simulink model "NoC_4x4x3"  (R2015a)
settings: Solver=ode45  StartTime=0.0  StopTime=10.0  RelTol=1e-3
undefined symbols (not defined in the file or in its folder): des, SELECT
undefined symbols (not defined in the file): MAX, MIN, T
libraries: simulink x48
(part 4 of 12)

== system NoC_4x4x3/Layer/PE00 ==
  Constant : Constant  Value=SELECT
  Create Generator Selection Variable : Subsystem  TreatAsAtomicUnit=on
      settings: PropExecContextOutsideSubsystem=on
  DST : EventBasedRandomNumber  Distribution=Arbitrary discrete  minUnid=1  maxUnid=16  numValueUnid=5  valueVecDisc=[1 2 3 4]  probVecDisc=[.25 .25 .25 .25]  Seed=SEED+5
  DST1 : EventBasedRandomNumber  Distribution=Arbitrary discrete  minUnid=1  maxUnid=16  numValueUnid=5  valueVecDisc=[1 2 3 4]  probVecDisc=[.25 .25 .25 .25]  Seed=SEED+50
  DST2 : EventBasedRandomNumber  Distribution=Arbitrary discrete  minUnid=1  maxUnid=16  numValueUnid=5  valueVecDisc=[1 2 3 4]  probVecDisc=[.25 .25 .25 .25]  Seed=SEED+500
  Enabled Gate : EnabledGate
  Entity Departure Event to Function-Call Event : EntityDepartureFunctionCallGenerator
  Entity Sink : EntitySink
  Entity Sink1 : EntitySink
  Generator 1 : TimeBasedEntityGenerator  Distribution=Exponential  Period=.1  InitialSeed=SEED+10  Maximum=.2  Mean=B  ResponseWhenUnblocked=Delayed restart  EntityType=Standard
  Infinite Server : InfiniteServer  ServiceTime=0  StatAverageWait=on
      settings: OutputPortMap=o4
  Input Switch : InputSwitch  SwitchingCriterion=From signal port p  StatNumberDeparted=on
  Loss : ToWorkspace  VariableName=Corner_Loss_Z2  SaveFormat=Timeseries  SampleTime=-1
  N : ToWorkspace  VariableName=Corner_N_Z2  SaveFormat=Timeseries  SampleTime=-1
  Read Timer : ReadTimer  TimerTag=Departure  StatAverageTimeElapsed=on
      settings: OutputPortMap=o3
  Router : ToWorkspace  VariableName=Corner_Mean_Z2  SaveFormat=Timeseries  SampleTime=-1
  Set Attribute : SetAttribute  AttributeName=DST_X|DST_Y|DST_Z  AttributeFrom=Signal port|Signal port|Signal port  AttributeValue=16|1|1  AttributeTreatAsVector=0|1|1  StatNumberDeparted=on  EvaluatedAttributeValue={ [];[];[]}
      settings: InputPortMap=u0,u1,u2
  Start Timer1 : StartTimer  TimerTag=Departure
  Time-Based Entity Generator : TimeBasedEntityGenerator  Distribution=Exponential  Period=15  InitialSeed=50510  Maximum=2  Mean=A  PriorityEntityGeneration=350  EntityType=Standard
  Time-Based Entity Generator1 : TimeBasedEntityGenerator  Period=REGULAR
  Time-Based Entity Generator2 : TimeBasedEntityGenerator  Distribution=Uniform  InitialSeed=56944  Minimum=MINU  Maximum=MAXU
  Data_out : PMIOPort  Port=1  Side=Right
  Data_in : PMIOPort  Port=2  Side=Left
  wires:
  Create Generator Selection Variable/1(Out1) -> Enabled Gate/1
  Entity Departure Event to Function-Call Event/1 -> Create Generator Selection Variable/Trigger
  Constant/1 -> Input Switch/1
  Read Timer/1 -> Router/1
  Input Switch/1 -> N/1
  DST/1 -> Set Attribute/1
  DST1/1 -> Set Attribute/2
  DST2/1 -> Set Attribute/3
  Infinite Server/1 -> Loss/1
  connections:
  Entity Departure Event to Function-Call Event/RConn1 -- Entity Sink/LConn1
  Time-Based Entity Generator/RConn1 -- Entity Departure Event to Function-Call Event/LConn1
  Generator 1/RConn1 -- Enabled Gate/LConn1
  Time-Based Entity Generator1/RConn1 -- Input Switch/LConn1
  Input Switch/LConn2 -- Time-Based Entity Generator2/RConn1
  Enabled Gate/RConn1 -- Input Switch/LConn3
  Start Timer1/LConn1 -- Set Attribute/RConn1
  Set Attribute/LConn1 -- Input Switch/RConn1
  Entity Sink1/LConn1 -- Read Timer/RConn1
  Data_in/RConn1 -- Read Timer/LConn1
  Start Timer1/RConn1 -- Infinite Server/LConn1
  Infinite Server/RConn1 -- Data_out/RConn1

== system NoC_4x4x3/Layer/PE01 ==
  Constant : Constant  Value=SELECT
  Create Generator Selection Variable : Subsystem  TreatAsAtomicUnit=on
      settings: PropExecContextOutsideSubsystem=on
  DST : EventBasedRandomNumber  Distribution=Arbitrary discrete  minUnid=1  maxUnid=16  numValueUnid=5  valueVecDisc=[1 2 3 4]  probVecDisc=[.25 .25 .25 .25]  Seed=SEED+5
  DST1 : EventBasedRandomNumber  Distribution=Arbitrary discrete  minUnid=1  maxUnid=16  numValueUnid=5  valueVecDisc=[1 2 3 4]  probVecDisc=[.25 .25 .25 .25]  Seed=SEED+50
  DST2 : EventBasedRandomNumber  Distribution=Arbitrary discrete  minUnid=1  maxUnid=16  numValueUnid=5  valueVecDisc=[1 2 3 4]  probVecDisc=[.25 .25 .25 .25]  Seed=SEED+500
  Enabled Gate : EnabledGate
  Entity Departure Event to Function-Call Event : EntityDepartureFunctionCallGenerator
  Entity Sink : EntitySink
  Entity Sink1 : EntitySink
  Generator 1 : TimeBasedEntityGenerator  Distribution=Exponential  Period=.1  InitialSeed=SEED+10  Maximum=.2  Mean=B  ResponseWhenUnblocked=Delayed restart  EntityType=Standard
  Infinite Server : InfiniteServer  ServiceTime=0  StatAverageWait=on
      settings: OutputPortMap=o4
  Input Switch : InputSwitch  SwitchingCriterion=From signal port p  StatNumberDeparted=on
  Loss : ToWorkspace  VariableName=Side_Loss_Z2  SaveFormat=Timeseries  SampleTime=-1
  N : ToWorkspace  VariableName=Side_N_Z2  SaveFormat=Timeseries  SampleTime=-1
  Read Timer : ReadTimer  TimerTag=Departure  StatAverageTimeElapsed=on
      settings: OutputPortMap=o3
  Router : ToWorkspace  VariableName=Side_Mean_Z2  SaveFormat=Timeseries  SampleTime=-1
  Set Attribute : SetAttribute  AttributeName=DST_X|DST_Y|DST_Z  AttributeFrom=Signal port|Signal port|Signal port  AttributeValue=16|1|1  AttributeTreatAsVector=0|1|1  StatNumberDeparted=on  EvaluatedAttributeValue={ [];[];[]}
      settings: InputPortMap=u0,u1,u2
  Start Timer : StartTimer  TimerTag=Departure
  Time-Based Entity Generator : TimeBasedEntityGenerator  Distribution=Exponential  Period=15  InitialSeed=60161  Maximum=2  Mean=A  PriorityEntityGeneration=350  EntityType=Standard
  Time-Based Entity Generator1 : TimeBasedEntityGenerator  Period=REGULAR
  Time-Based Entity Generator2 : TimeBasedEntityGenerator  Distribution=Uniform  InitialSeed=63378  Minimum=MINU  Maximum=MAXU
  Data_out : PMIOPort  Port=1  Side=Right
  Data_in : PMIOPort  Port=2  Side=Left
  wires:
  DST2/1 -> Set Attribute/3
  DST1/1 -> Set Attribute/2
  DST/1 -> Set Attribute/1
  Input Switch/1 -> N/1
  Read Timer/1 -> Router/1
  Constant/1 -> Input Switch/1
  Entity Departure Event to Function-Call Event/1 -> Create Generator Selection Variable/Trigger
  Create Generator Selection Variable/1(Out1) -> Enabled Gate/1
  Infinite Server/1 -> Loss/1
  connections:
  Data_in/RConn1 -- Read Timer/LConn1
  Entity Sink1/LConn1 -- Read Timer/RConn1
  Set Attribute/LConn1 -- Input Switch/RConn1
  Start Timer/LConn1 -- Set Attribute/RConn1
  Enabled Gate/RConn1 -- Input Switch/LConn3
  Input Switch/LConn2 -- Time-Based Entity Generator2/RConn1
  Time-Based Entity Generator1/RConn1 -- Input Switch/LConn1
  Generator 1/RConn1 -- Enabled Gate/LConn1
  Time-Based Entity Generator/RConn1 -- Entity Departure Event to Function-Call Event/LConn1
  Entity Departure Event to Function-Call Event/RConn1 -- Entity Sink/LConn1
  Start Timer/RConn1 -- Infinite Server/LConn1
  Infinite Server/RConn1 -- Data_out/RConn1

== system NoC_4x4x3/Layer/PE02 ==
  Cancel Timeout : CancelTimeout
  Constant : Constant  Value=SELECT
  Create Generator Selection Variable : Subsystem  TreatAsAtomicUnit=on
      settings: PropExecContextOutsideSubsystem=on
  DST : EventBasedRandomNumber  Distribution=Arbitrary discrete  minUnid=1  maxUnid=16  numValueUnid=5  valueVecDisc=[1 2 3 4]  probVecDisc=[.25 .25 .25 .25]  Seed=SEED+5
  DST1 : EventBasedRandomNumber  Distribution=Arbitrary discrete  minUnid=1  maxUnid=16  numValueUnid=5  valueVecDisc=[1 2 3 4]  probVecDisc=[.25 .25 .25 .25]  Seed=SEED+50
  DST2 : EventBasedRandomNumber  Distribution=Arbitrary discrete  minUnid=1  maxUnid=16  numValueUnid=5  valueVecDisc=[1 2 3 4]  probVecDisc=[.25 .25 .25 .25]  Seed=SEED+500
  Enabled Gate : EnabledGate
  Entity Departure Event to Function-Call Event : EntityDepartureFunctionCallGenerator
  Entity Sink : EntitySink
  Entity Sink1 : EntitySink
  Entity Sink2 : EntitySink
  Generator 1 : TimeBasedEntityGenerator  Distribution=Exponential  Period=.1  InitialSeed=SEED+10  Maximum=.2  Mean=B  ResponseWhenUnblocked=Delayed restart  EntityType=Standard
  Infinite Server : InfiniteServer  ServiceTime=D  EnableTOPort=on
  Input Switch : InputSwitch  SwitchingCriterion=From signal port p
  Schedule Timeout : ScheduleTimeout  TimeoutInterval=D
  Set Attribute : SetAttribute  AttributeName=DST_X|DST_Y|DST_Z  AttributeFrom=Signal port|Signal port|Signal port  AttributeValue=16|1|1  AttributeTreatAsVector=0|1|1  EvaluatedAttributeValue={ [];[];[]}
      settings: InputPortMap=u0,u1,u2
  Start Timer : StartTimer  TimerTag=Departure
  Time-Based Entity Generator : TimeBasedEntityGenerator  Distribution=Exponential  Period=15  InitialSeed=1059  Maximum=2  Mean=A  PriorityEntityGeneration=350  EntityType=Standard
  Time-Based Entity Generator1 : TimeBasedEntityGenerator  Period=REGULAR
  Time-Based Entity Generator2 : TimeBasedEntityGenerator  Distribution=Uniform  InitialSeed=4276  Minimum=MINU  Maximum=MAXU
  Data_out : PMIOPort  Port=1  Side=Right
  Data_in : PMIOPort  Port=2  Side=Left
  wires:
  DST2/1 -> Set Attribute/3
  DST1/1 -> Set Attribute/2
  DST/1 -> Set Attribute/1
  Constant/1 -> Input Switch/1
  Entity Departure Event to Function-Call Event/1 -> Create Generator Selection Variable/Trigger
  Create Generator Selection Variable/1(Out1) -> Enabled Gate/1
  connections:
  Infinite Server/RConn2 -- Entity Sink2/LConn1
  Schedule Timeout/RConn1 -- Infinite Server/LConn1
  Entity Sink1/LConn1 -- Data_in/RConn1
  Start Timer/LConn1 -- Cancel Timeout/RConn1
  Data_out/RConn1 -- Start Timer/RConn1
  Set Attribute/LConn1 -- Input Switch/RConn1
  Cancel Timeout/LConn1 -- Infinite Server/RConn1
  Schedule Timeout/LConn1 -- Set Attribute/RConn1
  Enabled Gate/RConn1 -- Input Switch/LConn3
  Input Switch/LConn2 -- Time-Based Entity Generator2/RConn1
  Time-Based Entity Generator1/RConn1 -- Input Switch/LConn1
  Generator 1/RConn1 -- Enabled Gate/LConn1
  Time-Based Entity Generator/RConn1 -- Entity Departure Event to Function-Call Event/LConn1
  Entity Departure Event to Function-Call Event/RConn1 -- Entity Sink/LConn1

== system NoC_4x4x3/Layer/PE03 ==
  Cancel Timeout : CancelTimeout
  Constant : Constant  Value=SELECT
  Create Generator Selection Variable : Subsystem  TreatAsAtomicUnit=on
      settings: PropExecContextOutsideSubsystem=on
  DST : EventBasedRandomNumber  Distribution=Arbitrary discrete  minUnid=1  maxUnid=16  numValueUnid=5  valueVecDisc=[1 2 3 4]  probVecDisc=[.25 .25 .25 .25]  Seed=SEED+5
  DST1 : EventBasedRandomNumber  Distribution=Arbitrary discrete  minUnid=1  maxUnid=16  numValueUnid=5  valueVecDisc=[1 2 3 4]  probVecDisc=[.25 .25 .25 .25]  Seed=SEED+50
  DST2 : EventBasedRandomNumber  Distribution=Arbitrary discrete  minUnid=1  maxUnid=16  numValueUnid=5  valueVecDisc=[1 2 3 4]  probVecDisc=[.25 .25 .25 .25]  Seed=SEED+500
  Enabled Gate : EnabledGate
  Entity Departure Event to Function-Call Event : EntityDepartureFunctionCallGenerator
  Entity Sink : EntitySink
  Entity Sink1 : EntitySink
  Entity Sink2 : EntitySink
  Generator 1 : TimeBasedEntityGenerator  Distribution=Exponential  Period=.1  InitialSeed=SEED+10  Maximum=.2  Mean=B  ResponseWhenUnblocked=Delayed restart  EntityType=Standard
  Infinite Server : InfiniteServer  ServiceTime=D  EnableTOPort=on
  Input Switch : InputSwitch  SwitchingCriterion=From signal port p
  Schedule Timeout : ScheduleTimeout  TimeoutInterval=D
  Set Attribute : SetAttribute  AttributeName=DST_X|DST_Y|DST_Z  AttributeFrom=Signal port|Signal port|Signal port  AttributeValue=16|1|1  AttributeTreatAsVector=0|1|1  EvaluatedAttributeValue={ [];[];[]}
      settings: InputPortMap=u0,u1,u2
  Start Timer : StartTimer  TimerTag=Departure
  Time-Based Entity Generator : TimeBasedEntityGenerator  Distribution=Exponential  Period=15  InitialSeed=7493  Maximum=2  Mean=A  PriorityEntityGeneration=350  EntityType=Standard
  Time-Based Entity Generator1 : TimeBasedEntityGenerator  Period=REGULAR
  Time-Based Entity Generator2 : TimeBasedEntityGenerator  Distribution=Uniform  InitialSeed=10710  Minimum=MINU  Maximum=MAXU
  Data_out : PMIOPort  Port=1  Side=Right
  Data_in : PMIOPort  Port=2  Side=Left
  wires:
  Create Generator Selection Variable/1(Out1) -> Enabled Gate/1
  Entity Departure Event to Function-Call Event/1 -> Create Generator Selection Variable/Trigger
  Constant/1 -> Input Switch/1
  DST/1 -> Set Attribute/1
  DST1/1 -> Set Attribute/2
  DST2/1 -> Set Attribute/3
  connections:
  Entity Departure Event to Function-Call Event/RConn1 -- Entity Sink/LConn1
  Time-Based Entity Generator/RConn1 -- Entity Departure Event to Function-Call Event/LConn1
  Generator 1/RConn1 -- Enabled Gate/LConn1
  Time-Based Entity Generator1/RConn1 -- Input Switch/LConn1
  Input Switch/LConn2 -- Time-Based Entity Generator2/RConn1
  Enabled Gate/RConn1 -- Input Switch/LConn3
  Schedule Timeout/LConn1 -- Set Attribute/RConn1
  Cancel Timeout/LConn1 -- Infinite Server/RConn1
  Set Attribute/LConn1 -- Input Switch/RConn1
  Data_out/RConn1 -- Start Timer/RConn1
  Start Timer/LConn1 -- Cancel Timeout/RConn1
  Entity Sink1/LConn1 -- Data_in/RConn1
  Schedule Timeout/RConn1 -- Infinite Server/LConn1
  Infinite Server/RConn2 -- Entity Sink2/LConn1

== system NoC_4x4x3/Layer/PE10 ==
  Cancel Timeout : CancelTimeout
  Constant : Constant  Value=SELECT
  Create Generator Selection Variable : Subsystem  TreatAsAtomicUnit=on
      settings: PropExecContextOutsideSubsystem=on
  DST : EventBasedRandomNumber  Distribution=Arbitrary discrete  minUnid=1  maxUnid=16  numValueUnid=5  valueVecDisc=[1 2 3 4]  probVecDisc=[.25 .25 .25 .25]  Seed=SEED+5
  DST1 : EventBasedRandomNumber  Distribution=Arbitrary discrete  minUnid=1  maxUnid=16  numValueUnid=5  valueVecDisc=[1 2 3 4]  probVecDisc=[.25 .25 .25 .25]  Seed=SEED+50
  DST2 : EventBasedRandomNumber  Distribution=Arbitrary discrete  minUnid=1  maxUnid=16  numValueUnid=5  valueVecDisc=[1 2 3 4]  probVecDisc=[.25 .25 .25 .25]  Seed=SEED+500
  Enabled Gate : EnabledGate
  Entity Departure Event to Function-Call Event : EntityDepartureFunctionCallGenerator
  Entity Sink : EntitySink
  Entity Sink1 : EntitySink
  Entity Sink2 : EntitySink
  Generator 1 : TimeBasedEntityGenerator  Distribution=Exponential  Period=.1  InitialSeed=SEED+10  Maximum=.2  Mean=B  ResponseWhenUnblocked=Delayed restart  EntityType=Standard
  Infinite Server : InfiniteServer  ServiceTime=D  EnableTOPort=on
  Input Switch : InputSwitch  SwitchingCriterion=From signal port p
  Schedule Timeout : ScheduleTimeout  TimeoutInterval=D
  Set Attribute : SetAttribute  AttributeName=DST_X|DST_Y|DST_Z  AttributeFrom=Signal port|Signal port|Signal port  AttributeValue=16|1|1  AttributeTreatAsVector=0|1|1  EvaluatedAttributeValue={ [];[];[]}
      settings: InputPortMap=u0,u1,u2
  Start Timer : StartTimer  TimerTag=Departure
  Time-Based Entity Generator : TimeBasedEntityGenerator  Distribution=Exponential  Period=15  InitialSeed=13927  Maximum=2  Mean=A  PriorityEntityGeneration=350  EntityType=Standard
  Time-Based Entity Generator1 : TimeBasedEntityGenerator  Period=REGULAR
  Time-Based Entity Generator2 : TimeBasedEntityGenerator  Distribution=Uniform  InitialSeed=17144  Minimum=MINU  Maximum=MAXU
  Data_out : PMIOPort  Port=1  Side=Right
  Data_in : PMIOPort  Port=2  Side=Left
  wires:
  DST2/1 -> Set Attribute/3
  DST1/1 -> Set Attribute/2
  DST/1 -> Set Attribute/1
  Constant/1 -> Input Switch/1
  Entity Departure Event to Function-Call Event/1 -> Create Generator Selection Variable/Trigger
  Create Generator Selection Variable/1(Out1) -> Enabled Gate/1
  connections:
  Infinite Server/RConn2 -- Entity Sink2/LConn1
  Schedule Timeout/RConn1 -- Infinite Server/LConn1
  Entity Sink1/LConn1 -- Data_in/RConn1
  Start Timer/LConn1 -- Cancel Timeout/RConn1
  Data_out/RConn1 -- Start Timer/RConn1
  Set Attribute/LConn1 -- Input Switch/RConn1
  Cancel Timeout/LConn1 -- Infinite Server/RConn1
  Schedule Timeout/LConn1 -- Set Attribute/RConn1
  Enabled Gate/RConn1 -- Input Switch/LConn3
  Input Switch/LConn2 -- Time-Based Entity Generator2/RConn1
  Time-Based Entity Generator1/RConn1 -- Input Switch/LConn1
  Generator 1/RConn1 -- Enabled Gate/LConn1
  Time-Based Entity Generator/RConn1 -- Entity Departure Event to Function-Call Event/LConn1
  Entity Departure Event to Function-Call Event/RConn1 -- Entity Sink/LConn1

== system NoC_4x4x3/Layer/PE11 ==
  Constant : Constant  Value=SELECT
  Create Generator Selection Variable : Subsystem  TreatAsAtomicUnit=on
      settings: PropExecContextOutsideSubsystem=on
  DST : EventBasedRandomNumber  Distribution=Arbitrary discrete  minUnid=1  maxUnid=16  numValueUnid=5  valueVecDisc=[1 2 3 4]  probVecDisc=[.25 .25 .25 .25]  Seed=SEED+5
  DST1 : EventBasedRandomNumber  Distribution=Arbitrary discrete  minUnid=1  maxUnid=16  numValueUnid=5  valueVecDisc=[1 2 3 4]  probVecDisc=[.25 .25 .25 .25]  Seed=SEED+50
  DST2 : EventBasedRandomNumber  Distribution=Arbitrary discrete  minUnid=1  maxUnid=16  numValueUnid=5  valueVecDisc=[1 2 3 4]  probVecDisc=[.25 .25 .25 .25]  Seed=SEED+500
  Enabled Gate : EnabledGate
  Entity Departure Event to Function-Call Event : EntityDepartureFunctionCallGenerator
  Entity Sink : EntitySink
  Entity Sink1 : EntitySink
  Generator 1 : TimeBasedEntityGenerator  Distribution=Exponential  Period=.1  InitialSeed=SEED+10  Maximum=.2  Mean=B  ResponseWhenUnblocked=Delayed restart  EntityType=Standard
  Infinite Server : InfiniteServer  ServiceTime=0  StatAverageWait=on
      settings: OutputPortMap=o4
  Input Switch : InputSwitch  SwitchingCriterion=From signal port p  StatNumberDeparted=on
  Loss : ToWorkspace  VariableName=Midlle_Loss_Z2  SaveFormat=Timeseries  SampleTime=-1
  N : ToWorkspace  VariableName=Midlle_N_Z2  SaveFormat=Timeseries  SampleTime=-1
  Read Timer : ReadTimer  TimerTag=Departure  StatAverageTimeElapsed=on
      settings: OutputPortMap=o3
  Router : ToWorkspace  VariableName=Midlle_Mean_Z2  SaveFormat=Timeseries  SampleTime=-1
  Set Attribute : SetAttribute  AttributeName=DST_X|DST_Y|DST_Z  AttributeFrom=Signal port|Signal port|Signal port  AttributeValue=16|1|1  AttributeTreatAsVector=0|1|1  StatNumberDeparted=on  EvaluatedAttributeValue={ [];[];[]}
      settings: InputPortMap=u0,u1,u2
  Start Timer : StartTimer  TimerTag=Departure
  Time-Based Entity Generator : TimeBasedEntityGenerator  Distribution=Exponential  Period=15  InitialSeed=20361  Maximum=2  Mean=A  PriorityEntityGeneration=350  EntityType=Standard
  Time-Based Entity Generator1 : TimeBasedEntityGenerator  Period=REGULAR
  Time-Based Entity Generator2 : TimeBasedEntityGenerator  Distribution=Uniform  InitialSeed=23578  Minimum=MINU  Maximum=MAXU
  Data_out : PMIOPort  Port=1  Side=Right
  Data_in : PMIOPort  Port=2  Side=Left
  wires:
  Create Generator Selection Variable/1(Out1) -> Enabled Gate/1
  Entity Departure Event to Function-Call Event/1 -> Create Generator Selection Variable/Trigger
  Constant/1 -> Input Switch/1
  Read Timer/1 -> Router/1
  Input Switch/1 -> N/1
  DST/1 -> Set Attribute/1
  DST1/1 -> Set Attribute/2
  DST2/1 -> Set Attribute/3
  Infinite Server/1 -> Loss/1
  connections:
  Entity Departure Event to Function-Call Event/RConn1 -- Entity Sink/LConn1
  Time-Based Entity Generator/RConn1 -- Entity Departure Event to Function-Call Event/LConn1
  Generator 1/RConn1 -- Enabled Gate/LConn1
  Time-Based Entity Generator1/RConn1 -- Input Switch/LConn1
  Input Switch/LConn2 -- Time-Based Entity Generator2/RConn1
  Enabled Gate/RConn1 -- Input Switch/LConn3
  Start Timer/LConn1 -- Set Attribute/RConn1
  Set Attribute/LConn1 -- Input Switch/RConn1
  Infinite Server/RConn1 -- Data_out/RConn1
  Entity Sink1/LConn1 -- Read Timer/RConn1
  Data_in/RConn1 -- Read Timer/LConn1
  Start Timer/RConn1 -- Infinite Server/LConn1

== system NoC_4x4x3/Layer/PE12 ==
  Cancel Timeout : CancelTimeout
  Constant : Constant  Value=SELECT
  Create Generator Selection Variable : Subsystem  TreatAsAtomicUnit=on
      settings: PropExecContextOutsideSubsystem=on
  DST : EventBasedRandomNumber  Distribution=Arbitrary discrete  minUnid=1  maxUnid=16  numValueUnid=5  valueVecDisc=[1 2 3 4]  probVecDisc=[.25 .25 .25 .25]  Seed=SEED+5
  DST1 : EventBasedRandomNumber  Distribution=Arbitrary discrete  minUnid=1  maxUnid=16  numValueUnid=5  valueVecDisc=[1 2 3 4]  probVecDisc=[.25 .25 .25 .25]  Seed=SEED+50
  DST2 : EventBasedRandomNumber  Distribution=Arbitrary discrete  minUnid=1  maxUnid=16  numValueUnid=5  valueVecDisc=[1 2 3 4]  probVecDisc=[.25 .25 .25 .25]  Seed=SEED+500
  Enabled Gate : EnabledGate
  Entity Departure Event to Function-Call Event : EntityDepartureFunctionCallGenerator
  Entity Sink : EntitySink
  Entity Sink1 : EntitySink
  Entity Sink2 : EntitySink
  Generator 1 : TimeBasedEntityGenerator  Distribution=Exponential  Period=.1  InitialSeed=SEED+10  Maximum=.2  Mean=B  ResponseWhenUnblocked=Delayed restart  EntityType=Standard
  Infinite Server : InfiniteServer  ServiceTime=D  EnableTOPort=on
  Input Switch : InputSwitch  SwitchingCriterion=From signal port p
  Schedule Timeout : ScheduleTimeout  TimeoutInterval=D
  Set Attribute : SetAttribute  AttributeName=DST_X|DST_Y|DST_Z  AttributeFrom=Signal port|Signal port|Signal port  AttributeValue=16|1|1  AttributeTreatAsVector=0|1|1  EvaluatedAttributeValue={ [];[];[]}
      settings: InputPortMap=u0,u1,u2
  Start Timer : StartTimer  TimerTag=Departure
  Time-Based Entity Generator : TimeBasedEntityGenerator  Distribution=Exponential  Period=15  InitialSeed=26795  Maximum=2  Mean=A  PriorityEntityGeneration=350  EntityType=Standard
  Time-Based Entity Generator1 : TimeBasedEntityGenerator  Period=REGULAR
  Time-Based Entity Generator2 : TimeBasedEntityGenerator  Distribution=Uniform  InitialSeed=30012  Minimum=MINU  Maximum=MAXU
  Data_out : PMIOPort  Port=1  Side=Right
  Data_in : PMIOPort  Port=2  Side=Left
  wires:
  Create Generator Selection Variable/1(Out1) -> Enabled Gate/1
  Entity Departure Event to Function-Call Event/1 -> Create Generator Selection Variable/Trigger
  Constant/1 -> Input Switch/1
  DST/1 -> Set Attribute/1
  DST1/1 -> Set Attribute/2
  DST2/1 -> Set Attribute/3
  connections:
  Entity Departure Event to Function-Call Event/RConn1 -- Entity Sink/LConn1
  Time-Based Entity Generator/RConn1 -- Entity Departure Event to Function-Call Event/LConn1
  Generator 1/RConn1 -- Enabled Gate/LConn1
  Time-Based Entity Generator1/RConn1 -- Input Switch/LConn1
  Input Switch/LConn2 -- Time-Based Entity Generator2/RConn1
  Enabled Gate/RConn1 -- Input Switch/LConn3
  Schedule Timeout/LConn1 -- Set Attribute/RConn1
  Cancel Timeout/LConn1 -- Infinite Server/RConn1
  Set Attribute/LConn1 -- Input Switch/RConn1
  Data_out/RConn1 -- Start Timer/RConn1
  Start Timer/LConn1 -- Cancel Timeout/RConn1
  Entity Sink1/LConn1 -- Data_in/RConn1
  Schedule Timeout/RConn1 -- Infinite Server/LConn1
  Infinite Server/RConn2 -- Entity Sink2/LConn1

== system NoC_4x4x3/Layer/PE13 ==
  Cancel Timeout : CancelTimeout
  Constant : Constant  Value=SELECT
  Create Generator Selection Variable : Subsystem  TreatAsAtomicUnit=on
      settings: PropExecContextOutsideSubsystem=on
  DST : EventBasedRandomNumber  Distribution=Arbitrary discrete  minUnid=1  maxUnid=16  numValueUnid=5  valueVecDisc=[1 2 3 4]  probVecDisc=[.25 .25 .25 .25]  Seed=SEED+5
  DST1 : EventBasedRandomNumber  Distribution=Arbitrary discrete  minUnid=1  maxUnid=16  numValueUnid=5  valueVecDisc=[1 2 3 4]  probVecDisc=[.25 .25 .25 .25]  Seed=SEED+50
  DST2 : EventBasedRandomNumber  Distribution=Arbitrary discrete  minUnid=1  maxUnid=16  numValueUnid=5  valueVecDisc=[1 2 3 4]  probVecDisc=[.25 .25 .25 .25]  Seed=SEED+500
  Enabled Gate : EnabledGate
  Entity Departure Event to Function-Call Event : EntityDepartureFunctionCallGenerator
  Entity Sink : EntitySink
  Entity Sink1 : EntitySink
  Entity Sink2 : EntitySink
  Generator 1 : TimeBasedEntityGenerator  Distribution=Exponential  Period=.1  InitialSeed=SEED+10  Maximum=.2  Mean=B  ResponseWhenUnblocked=Delayed restart  EntityType=Standard
  Infinite Server : InfiniteServer  ServiceTime=D  EnableTOPort=on
  Input Switch : InputSwitch  SwitchingCriterion=From signal port p
  Schedule Timeout : ScheduleTimeout  TimeoutInterval=D
  Set Attribute : SetAttribute  AttributeName=DST_X|DST_Y|DST_Z  AttributeFrom=Signal port|Signal port|Signal port  AttributeValue=16|1|1  AttributeTreatAsVector=0|1|1  EvaluatedAttributeValue={ [];[];[]}
      settings: InputPortMap=u0,u1,u2
  Start Timer : StartTimer  TimerTag=Departure
  Time-Based Entity Generator : TimeBasedEntityGenerator  Distribution=Exponential  Period=15  InitialSeed=33229  Maximum=2  Mean=A  PriorityEntityGeneration=350  EntityType=Standard
  Time-Based Entity Generator1 : TimeBasedEntityGenerator  Period=REGULAR
  Time-Based Entity Generator2 : TimeBasedEntityGenerator  Distribution=Uniform  InitialSeed=36446  Minimum=MINU  Maximum=MAXU
  Data_out : PMIOPort  Port=1  Side=Right
  Data_in : PMIOPort  Port=2  Side=Left
  wires:
  DST2/1 -> Set Attribute/3
  DST1/1 -> Set Attribute/2
  DST/1 -> Set Attribute/1
  Constant/1 -> Input Switch/1
  Entity Departure Event to Function-Call Event/1 -> Create Generator Selection Variable/Trigger
  Create Generator Selection Variable/1(Out1) -> Enabled Gate/1
  connections:
  Infinite Server/RConn2 -- Entity Sink2/LConn1
  Schedule Timeout/RConn1 -- Infinite Server/LConn1
  Entity Sink1/LConn1 -- Data_in/RConn1
  Start Timer/LConn1 -- Cancel Timeout/RConn1
  Data_out/RConn1 -- Start Timer/RConn1
  Set Attribute/LConn1 -- Input Switch/RConn1
  Cancel Timeout/LConn1 -- Infinite Server/RConn1
  Schedule Timeout/LConn1 -- Set Attribute/RConn1
  Enabled Gate/RConn1 -- Input Switch/LConn3
  Input Switch/LConn2 -- Time-Based Entity Generator2/RConn1
  Time-Based Entity Generator1/RConn1 -- Input Switch/LConn1
  Generator 1/RConn1 -- Enabled Gate/LConn1
  Time-Based Entity Generator/RConn1 -- Entity Departure Event to Function-Call Event/LConn1
  Entity Departure Event to Function-Call Event/RConn1 -- Entity Sink/LConn1

== system NoC_4x4x3/Layer/PE20 ==
  Cancel Timeout : CancelTimeout
  Constant : Constant  Value=SELECT
  Create Generator Selection Variable : Subsystem  TreatAsAtomicUnit=on
      settings: PropExecContextOutsideSubsystem=on
  DST : EventBasedRandomNumber  Distribution=Arbitrary discrete  minUnid=1  maxUnid=16  numValueUnid=5  valueVecDisc=[1 2 3 4]  probVecDisc=[.25 .25 .25 .25]  Seed=SEED+5
  DST1 : EventBasedRandomNumber  Distribution=Arbitrary discrete  minUnid=1  maxUnid=16  numValueUnid=5  valueVecDisc=[1 2 3 4]  probVecDisc=[.25 .25 .25 .25]  Seed=SEED+50
  DST2 : EventBasedRandomNumber  Distribution=Arbitrary discrete  minUnid=1  maxUnid=16  numValueUnid=5  valueVecDisc=[1 2 3 4]  probVecDisc=[.25 .25 .25 .25]  Seed=SEED+500
  Enabled Gate : EnabledGate
  Entity Departure Event to Function-Call Event : EntityDepartureFunctionCallGenerator
  Entity Sink : EntitySink
  Entity Sink1 : EntitySink
  Entity Sink2 : EntitySink
  Generator 1 : TimeBasedEntityGenerator  Distribution=Exponential  Period=.1  InitialSeed=SEED+10  Maximum=.2  Mean=B  ResponseWhenUnblocked=Delayed restart  EntityType=Standard
  Infinite Server : InfiniteServer  ServiceTime=D  EnableTOPort=on
  Input Switch : InputSwitch  SwitchingCriterion=From signal port p
  Schedule Timeout : ScheduleTimeout  TimeoutInterval=D
  Set Attribute : SetAttribute  AttributeName=DST_X|DST_Y|DST_Z  AttributeFrom=Signal port|Signal port|Signal port  AttributeValue=16|1|1  AttributeTreatAsVector=0|1|1  EvaluatedAttributeValue={ [];[];[]}
      settings: InputPortMap=u0,u1,u2
  Start Timer : StartTimer  TimerTag=Departure
  Time-Based Entity Generator : TimeBasedEntityGenerator  Distribution=Exponential  Period=15  InitialSeed=39663  Maximum=2  Mean=A  PriorityEntityGeneration=350  EntityType=Standard
  Time-Based Entity Generator1 : TimeBasedEntityGenerator  Period=REGULAR
  Time-Based Entity Generator2 : TimeBasedEntityGenerator  Distribution=Uniform  InitialSeed=42880  Minimum=MINU  Maximum=MAXU
  Data_out : PMIOPort  Port=1  Side=Right
  Data_in : PMIOPort  Port=2  Side=Left
  wires:
  Create Generator Selection Variable/1(Out1) -> Enabled Gate/1
  Entity Departure Event to Function-Call Event/1 -> Create Generator Selection Variable/Trigger
  Constant/1 -> Input Switch/1
  DST/1 -> Set Attribute/1
  DST1/1 -> Set Attribute/2
  DST2/1 -> Set Attribute/3
  connections:
  Entity Departure Event to Function-Call Event/RConn1 -- Entity Sink/LConn1
  Time-Based Entity Generator/RConn1 -- Entity Departure Event to Function-Call Event/LConn1
  Generator 1/RConn1 -- Enabled Gate/LConn1
  Time-Based Entity Generator1/RConn1 -- Input Switch/LConn1
  Input Switch/LConn2 -- Time-Based Entity Generator2/RConn1
  Enabled Gate/RConn1 -- Input Switch/LConn3
  Schedule Timeout/LConn1 -- Set Attribute/RConn1
  Cancel Timeout/LConn1 -- Infinite Server/RConn1
  Set Attribute/LConn1 -- Input Switch/RConn1
  Data_out/RConn1 -- Start Timer/RConn1
  Start Timer/LConn1 -- Cancel Timeout/RConn1
  Entity Sink1/LConn1 -- Data_in/RConn1
  Schedule Timeout/RConn1 -- Infinite Server/LConn1
  Infinite Server/RConn2 -- Entity Sink2/LConn1

== system NoC_4x4x3/Layer/PE21 ==
  Cancel Timeout : CancelTimeout
  Constant : Constant  Value=SELECT
  Create Generator Selection Variable : Subsystem  TreatAsAtomicUnit=on
      settings: PropExecContextOutsideSubsystem=on
  DST : EventBasedRandomNumber  Distribution=Arbitrary discrete  minUnid=1  maxUnid=16  numValueUnid=5  valueVecDisc=[1 2 3 4]  probVecDisc=[.25 .25 .25 .25]  Seed=SEED+5
  DST1 : EventBasedRandomNumber  Distribution=Arbitrary discrete  minUnid=1  maxUnid=16  numValueUnid=5  valueVecDisc=[1 2 3 4]  probVecDisc=[.25 .25 .25 .25]  Seed=SEED+50
  DST2 : EventBasedRandomNumber  Distribution=Arbitrary discrete  minUnid=1  maxUnid=16  numValueUnid=5  valueVecDisc=[1 2 3 4]  probVecDisc=[.25 .25 .25 .25]  Seed=SEED+500
  Enabled Gate : EnabledGate
  Entity Departure Event to Function-Call Event : EntityDepartureFunctionCallGenerator
  Entity Sink : EntitySink
  Entity Sink1 : EntitySink
  Entity Sink2 : EntitySink
  Generator 1 : TimeBasedEntityGenerator  Distribution=Exponential  Period=.1  InitialSeed=SEED+10  Maximum=.2  Mean=B  ResponseWhenUnblocked=Delayed restart  EntityType=Standard
  Infinite Server : InfiniteServer  ServiceTime=D  EnableTOPort=on
  Input Switch : InputSwitch  SwitchingCriterion=From signal port p
  Schedule Timeout : ScheduleTimeout  TimeoutInterval=D
  Set Attribute : SetAttribute  AttributeName=DST_X|DST_Y|DST_Z  AttributeFrom=Signal port|Signal port|Signal port  AttributeValue=16|1|1  AttributeTreatAsVector=0|1|1  EvaluatedAttributeValue={ [];[];[]}
      settings: InputPortMap=u0,u1,u2
  Start Timer : StartTimer  TimerTag=Departure
  Time-Based Entity Generator : TimeBasedEntityGenerator  Distribution=Exponential  Period=15  InitialSeed=46097  Maximum=2  Mean=A  PriorityEntityGeneration=350  EntityType=Standard
  Time-Based Entity Generator1 : TimeBasedEntityGenerator  Period=REGULAR
  Time-Based Entity Generator2 : TimeBasedEntityGenerator  Distribution=Uniform  InitialSeed=49314  Minimum=MINU  Maximum=MAXU
  Data_out : PMIOPort  Port=1  Side=Right
  Data_in : PMIOPort  Port=2  Side=Left
  wires:
  DST2/1 -> Set Attribute/3
  DST1/1 -> Set Attribute/2
  DST/1 -> Set Attribute/1
  Constant/1 -> Input Switch/1
  Entity Departure Event to Function-Call Event/1 -> Create Generator Selection Variable/Trigger
  Create Generator Selection Variable/1(Out1) -> Enabled Gate/1
  connections:
  Infinite Server/RConn2 -- Entity Sink2/LConn1
  Schedule Timeout/RConn1 -- Infinite Server/LConn1
  Entity Sink1/LConn1 -- Data_in/RConn1
  Start Timer/LConn1 -- Cancel Timeout/RConn1
  Data_out/RConn1 -- Start Timer/RConn1
  Set Attribute/LConn1 -- Input Switch/RConn1
  Cancel Timeout/LConn1 -- Infinite Server/RConn1
  Schedule Timeout/LConn1 -- Set Attribute/RConn1
  Enabled Gate/RConn1 -- Input Switch/LConn3
  Input Switch/LConn2 -- Time-Based Entity Generator2/RConn1
  Time-Based Entity Generator1/RConn1 -- Input Switch/LConn1
  Generator 1/RConn1 -- Enabled Gate/LConn1
  Time-Based Entity Generator/RConn1 -- Entity Departure Event to Function-Call Event/LConn1
  Entity Departure Event to Function-Call Event/RConn1 -- Entity Sink/LConn1

== system NoC_4x4x3/Layer/PE22 ==
  Cancel Timeout : CancelTimeout
  Constant : Constant  Value=SELECT
  Create Generator Selection Variable : Subsystem  TreatAsAtomicUnit=on
      settings: PropExecContextOutsideSubsystem=on
  DST : EventBasedRandomNumber  Distribution=Arbitrary discrete  minUnid=1  maxUnid=16  numValueUnid=5  valueVecDisc=[1 2 3 4]  probVecDisc=[.25 .25 .25 .25]  Seed=SEED+5
  DST1 : EventBasedRandomNumber  Distribution=Arbitrary discrete  minUnid=1  maxUnid=16  numValueUnid=5  valueVecDisc=[1 2 3 4]  probVecDisc=[.25 .25 .25 .25]  Seed=SEED+50
  DST2 : EventBasedRandomNumber  Distribution=Arbitrary discrete  minUnid=1  maxUnid=16  numValueUnid=5  valueVecDisc=[1 2 3 4]  probVecDisc=[.25 .25 .25 .25]  Seed=SEED+500
  Enabled Gate : EnabledGate
  Entity Departure Event to Function-Call Event : EntityDepartureFunctionCallGenerator
  Entity Sink : EntitySink
  Entity Sink1 : EntitySink
  Entity Sink2 : EntitySink
  Generator 1 : TimeBasedEntityGenerator  Distribution=Exponential  Period=.1  InitialSeed=SEED+10  Maximum=.2  Mean=B  ResponseWhenUnblocked=Delayed restart  EntityType=Standard
  Infinite Server : InfiniteServer  ServiceTime=D  EnableTOPort=on
  Input Switch : InputSwitch  SwitchingCriterion=From signal port p
  Schedule Timeout : ScheduleTimeout  TimeoutInterval=D
  Set Attribute : SetAttribute  AttributeName=DST_X|DST_Y|DST_Z  AttributeFrom=Signal port|Signal port|Signal port  AttributeValue=16|1|1  AttributeTreatAsVector=0|1|1  EvaluatedAttributeValue={ [];[];[]}
      settings: InputPortMap=u0,u1,u2
  Start Timer : StartTimer  TimerTag=Departure
  Time-Based Entity Generator : TimeBasedEntityGenerator  Distribution=Exponential  Period=15  InitialSeed=52531  Maximum=2  Mean=A  PriorityEntityGeneration=350  EntityType=Standard
  Time-Based Entity Generator1 : TimeBasedEntityGenerator  Period=REGULAR
  Time-Based Entity Generator2 : TimeBasedEntityGenerator  Distribution=Uniform  InitialSeed=55748  Minimum=MINU  Maximum=MAXU
  Data_out : PMIOPort  Port=1  Side=Right
  Data_in : PMIOPort  Port=2  Side=Left
  wires:
  DST2/1 -> Set Attribute/3
  DST1/1 -> Set Attribute/2
  DST/1 -> Set Attribute/1
  Constant/1 -> Input Switch/1
  Entity Departure Event to Function-Call Event/1 -> Create Generator Selection Variable/Trigger
  Create Generator Selection Variable/1(Out1) -> Enabled Gate/1
  connections:
  Infinite Server/RConn2 -- Entity Sink2/LConn1
  Schedule Timeout/RConn1 -- Infinite Server/LConn1
  Entity Sink1/LConn1 -- Data_in/RConn1
  Start Timer/LConn1 -- Cancel Timeout/RConn1
  Data_out/RConn1 -- Start Timer/RConn1
  Set Attribute/LConn1 -- Input Switch/RConn1
  Cancel Timeout/LConn1 -- Infinite Server/RConn1
  Schedule Timeout/LConn1 -- Set Attribute/RConn1
  Enabled Gate/RConn1 -- Input Switch/LConn3
  Input Switch/LConn2 -- Time-Based Entity Generator2/RConn1
  Time-Based Entity Generator1/RConn1 -- Input Switch/LConn1
  Generator 1/RConn1 -- Enabled Gate/LConn1
  Time-Based Entity Generator/RConn1 -- Entity Departure Event to Function-Call Event/LConn1
  Entity Departure Event to Function-Call Event/RConn1 -- Entity Sink/LConn1

== system NoC_4x4x3/Layer/PE23 ==
  Cancel Timeout : CancelTimeout
  Constant : Constant  Value=SELECT
  Create Generator Selection Variable : Subsystem  TreatAsAtomicUnit=on
      settings: PropExecContextOutsideSubsystem=on
  DST : EventBasedRandomNumber  Distribution=Arbitrary discrete  minUnid=1  maxUnid=16  numValueUnid=5  valueVecDisc=[1 2 3 4]  probVecDisc=[.25 .25 .25 .25]  Seed=SEED+5
  DST1 : EventBasedRandomNumber  Distribution=Arbitrary discrete  minUnid=1  maxUnid=16  numValueUnid=5  valueVecDisc=[1 2 3 4]  probVecDisc=[.25 .25 .25 .25]  Seed=SEED+50
  DST2 : EventBasedRandomNumber  Distribution=Arbitrary discrete  minUnid=1  maxUnid=16  numValueUnid=5  valueVecDisc=[1 2 3 4]  probVecDisc=[.25 .25 .25 .25]  Seed=SEED+500
  Enabled Gate : EnabledGate
  Entity Departure Event to Function-Call Event : EntityDepartureFunctionCallGenerator
  Entity Sink : EntitySink
  Entity Sink1 : EntitySink
  Entity Sink2 : EntitySink
  Generator 1 : TimeBasedEntityGenerator  Distribution=Exponential  Period=.1  InitialSeed=SEED+10  Maximum=.2  Mean=B  ResponseWhenUnblocked=Delayed restart  EntityType=Standard
  Infinite Server : InfiniteServer  ServiceTime=D  EnableTOPort=on
  Input Switch : InputSwitch  SwitchingCriterion=From signal port p
  Schedule Timeout : ScheduleTimeout  TimeoutInterval=D
  Set Attribute : SetAttribute  AttributeName=DST_X|DST_Y|DST_Z  AttributeFrom=Signal port|Signal port|Signal port  AttributeValue=16|1|1  AttributeTreatAsVector=0|1|1  EvaluatedAttributeValue={ [];[];[]}
      settings: InputPortMap=u0,u1,u2
  Start Timer : StartTimer  TimerTag=Departure
  Time-Based Entity Generator : TimeBasedEntityGenerator  Distribution=Exponential  Period=15  InitialSeed=58965  Maximum=2  Mean=A  PriorityEntityGeneration=350  EntityType=Standard
  Time-Based Entity Generator1 : TimeBasedEntityGenerator  Period=REGULAR
  Time-Based Entity Generator2 : TimeBasedEntityGenerator  Distribution=Uniform  InitialSeed=62182  Minimum=MINU  Maximum=MAXU
  Data_out : PMIOPort  Port=1  Side=Right
  Data_in : PMIOPort  Port=2  Side=Left
  wires:
  Create Generator Selection Variable/1(Out1) -> Enabled Gate/1
  Entity Departure Event to Function-Call Event/1 -> Create Generator Selection Variable/Trigger
  Constant/1 -> Input Switch/1
  DST/1 -> Set Attribute/1
  DST1/1 -> Set Attribute/2
  DST2/1 -> Set Attribute/3
  connections:
  Entity Departure Event to Function-Call Event/RConn1 -- Entity Sink/LConn1
  Time-Based Entity Generator/RConn1 -- Entity Departure Event to Function-Call Event/LConn1
  Generator 1/RConn1 -- Enabled Gate/LConn1
  Time-Based Entity Generator1/RConn1 -- Input Switch/LConn1
  Input Switch/LConn2 -- Time-Based Entity Generator2/RConn1
  Enabled Gate/RConn1 -- Input Switch/LConn3
  Schedule Timeout/LConn1 -- Set Attribute/RConn1
  Cancel Timeout/LConn1 -- Infinite Server/RConn1
  Set Attribute/LConn1 -- Input Switch/RConn1
  Data_out/RConn1 -- Start Timer/RConn1
  Start Timer/LConn1 -- Cancel Timeout/RConn1
  Entity Sink1/LConn1 -- Data_in/RConn1
  Schedule Timeout/RConn1 -- Infinite Server/LConn1
  Infinite Server/RConn2 -- Entity Sink2/LConn1

== system NoC_4x4x3/Layer/PE30 ==
  Cancel Timeout : CancelTimeout
  Constant : Constant  Value=SELECT
  Create Generator Selection Variable : Subsystem  TreatAsAtomicUnit=on
      settings: PropExecContextOutsideSubsystem=on
  DST : EventBasedRandomNumber  Distribution=Arbitrary discrete  minUnid=1  maxUnid=16  numValueUnid=5  valueVecDisc=[1 2 3 4]  probVecDisc=[.25 .25 .25 .25]  Seed=SEED+5
  DST1 : EventBasedRandomNumber  Distribution=Arbitrary discrete  minUnid=1  maxUnid=16  numValueUnid=5  valueVecDisc=[1 2 3 4]  probVecDisc=[.25 .25 .25 .25]  Seed=SEED+50
  DST2 : EventBasedRandomNumber  Distribution=Arbitrary discrete  minUnid=1  maxUnid=16  numValueUnid=5  valueVecDisc=[1 2 3 4]  probVecDisc=[.25 .25 .25 .25]  Seed=SEED+500
  Enabled Gate : EnabledGate
  Entity Departure Event to Function-Call Event : EntityDepartureFunctionCallGenerator
  Entity Sink : EntitySink
  Entity Sink1 : EntitySink
  Entity Sink2 : EntitySink
  Generator 1 : TimeBasedEntityGenerator  Distribution=Exponential  Period=.1  InitialSeed=SEED+10  Maximum=.2  Mean=B  ResponseWhenUnblocked=Delayed restart  EntityType=Standard
  Infinite Server : InfiniteServer  ServiceTime=D  EnableTOPort=on
  Input Switch : InputSwitch  SwitchingCriterion=From signal port p
  Schedule Timeout : ScheduleTimeout  TimeoutInterval=D
  Set Attribute : SetAttribute  AttributeName=DST_X|DST_Y|DST_Z  AttributeFrom=Signal port|Signal port|Signal port  AttributeValue=16|1|1  AttributeTreatAsVector=0|1|1  EvaluatedAttributeValue={ [];[];[]}
      settings: InputPortMap=u0,u1,u2
  Start Timer : StartTimer  TimerTag=Departure
  Time-Based Entity Generator : TimeBasedEntityGenerator  Distribution=Exponential  Period=15  InitialSeed=65399  Maximum=2  Mean=A  PriorityEntityGeneration=350  EntityType=Standard
  Time-Based Entity Generator1 : TimeBasedEntityGenerator  Period=REGULAR
  Time-Based Entity Generator2 : TimeBasedEntityGenerator  Distribution=Uniform  InitialSeed=3080  Minimum=MINU  Maximum=MAXU
  Data_out : PMIOPort  Port=1  Side=Right
  Data_in : PMIOPort  Port=2  Side=Left
  wires:
  DST2/1 -> Set Attribute/3
  DST1/1 -> Set Attribute/2
  DST/1 -> Set Attribute/1
  Constant/1 -> Input Switch/1
  Entity Departure Event to Function-Call Event/1 -> Create Generator Selection Variable/Trigger
  Create Generator Selection Variable/1(Out1) -> Enabled Gate/1
  connections:
  Infinite Server/RConn2 -- Entity Sink2/LConn1
  Schedule Timeout/RConn1 -- Infinite Server/LConn1
  Entity Sink1/LConn1 -- Data_in/RConn1
  Start Timer/LConn1 -- Cancel Timeout/RConn1
  Data_out/RConn1 -- Start Timer/RConn1
  Set Attribute/LConn1 -- Input Switch/RConn1
  Cancel Timeout/LConn1 -- Infinite Server/RConn1
  Schedule Timeout/LConn1 -- Set Attribute/RConn1
  Enabled Gate/RConn1 -- Input Switch/LConn3
  Input Switch/LConn2 -- Time-Based Entity Generator2/RConn1
  Time-Based Entity Generator1/RConn1 -- Input Switch/LConn1
  Generator 1/RConn1 -- Enabled Gate/LConn1
  Time-Based Entity Generator/RConn1 -- Entity Departure Event to Function-Call Event/LConn1
  Entity Departure Event to Function-Call Event/RConn1 -- Entity Sink/LConn1

== system NoC_4x4x3/Layer/PE31 ==
  Cancel Timeout : CancelTimeout
  Constant : Constant  Value=SELECT
  Create Generator Selection Variable : Subsystem  TreatAsAtomicUnit=on
      settings: PropExecContextOutsideSubsystem=on
  DST : EventBasedRandomNumber  Distribution=Arbitrary discrete  minUnid=1  maxUnid=16  numValueUnid=5  valueVecDisc=[1 2 3 4]  probVecDisc=[.25 .25 .25 .25]  Seed=SEED+5
  DST1 : EventBasedRandomNumber  Distribution=Arbitrary discrete  minUnid=1  maxUnid=16  numValueUnid=5  valueVecDisc=[1 2 3 4]  probVecDisc=[.25 .25 .25 .25]  Seed=SEED+50
  DST2 : EventBasedRandomNumber  Distribution=Arbitrary discrete  minUnid=1  maxUnid=16  numValueUnid=5  valueVecDisc=[1 2 3 4]  probVecDisc=[.25 .25 .25 .25]  Seed=SEED+500
  Enabled Gate : EnabledGate
  Entity Departure Event to Function-Call Event : EntityDepartureFunctionCallGenerator
  Entity Sink : EntitySink
  Entity Sink1 : EntitySink
  Entity Sink2 : EntitySink
  Generator 1 : TimeBasedEntityGenerator  Distribution=Exponential  Period=.1  InitialSeed=SEED+10  Maximum=.2  Mean=B  ResponseWhenUnblocked=Delayed restart  EntityType=Standard
  Infinite Server : InfiniteServer  ServiceTime=D  EnableTOPort=on
  Input Switch : InputSwitch  SwitchingCriterion=From signal port p
  Schedule Timeout : ScheduleTimeout  TimeoutInterval=D
  Set Attribute : SetAttribute  AttributeName=DST_X|DST_Y|DST_Z  AttributeFrom=Signal port|Signal port|Signal port  AttributeValue=16|1|1  AttributeTreatAsVector=0|1|1  EvaluatedAttributeValue={ [];[];[]}
      settings: InputPortMap=u0,u1,u2
  Start Timer : StartTimer  TimerTag=Departure
  Time-Based Entity Generator : TimeBasedEntityGenerator  Distribution=Exponential  Period=15  InitialSeed=6297  Maximum=2  Mean=A  PriorityEntityGeneration=350  EntityType=Standard
  Time-Based Entity Generator1 : TimeBasedEntityGenerator  Period=REGULAR
  Time-Based Entity Generator2 : TimeBasedEntityGenerator  Distribution=Uniform  InitialSeed=9514  Minimum=MINU  Maximum=MAXU
  Data_out : PMIOPort  Port=1  Side=Right
  Data_in : PMIOPort  Port=2  Side=Left
  wires:
  Create Generator Selection Variable/1(Out1) -> Enabled Gate/1
  Entity Departure Event to Function-Call Event/1 -> Create Generator Selection Variable/Trigger
  Constant/1 -> Input Switch/1
  DST/1 -> Set Attribute/1
  DST1/1 -> Set Attribute/2
  DST2/1 -> Set Attribute/3
  connections:
  Entity Departure Event to Function-Call Event/RConn1 -- Entity Sink/LConn1
  Time-Based Entity Generator/RConn1 -- Entity Departure Event to Function-Call Event/LConn1
  Generator 1/RConn1 -- Enabled Gate/LConn1
  Time-Based Entity Generator1/RConn1 -- Input Switch/LConn1
  Input Switch/LConn2 -- Time-Based Entity Generator2/RConn1
  Enabled Gate/RConn1 -- Input Switch/LConn3
  Schedule Timeout/LConn1 -- Set Attribute/RConn1
  Cancel Timeout/LConn1 -- Infinite Server/RConn1
  Set Attribute/LConn1 -- Input Switch/RConn1
  Data_out/RConn1 -- Start Timer/RConn1
  Start Timer/LConn1 -- Cancel Timeout/RConn1
  Entity Sink1/LConn1 -- Data_in/RConn1
  Schedule Timeout/RConn1 -- Infinite Server/LConn1
  Infinite Server/RConn2 -- Entity Sink2/LConn1

== system NoC_4x4x3/Layer/PE32 ==
  Cancel Timeout : CancelTimeout
  Constant : Constant  Value=SELECT
  Create Generator Selection Variable : Subsystem  TreatAsAtomicUnit=on
      settings: PropExecContextOutsideSubsystem=on
  DST : EventBasedRandomNumber  Distribution=Arbitrary discrete  minUnid=1  maxUnid=16  numValueUnid=5  valueVecDisc=[1 2 3 4]  probVecDisc=[.25 .25 .25 .25]  Seed=SEED+5
  DST1 : EventBasedRandomNumber  Distribution=Arbitrary discrete  minUnid=1  maxUnid=16  numValueUnid=5  valueVecDisc=[1 2 3 4]  probVecDisc=[.25 .25 .25 .25]  Seed=SEED+50
  DST2 : EventBasedRandomNumber  Distribution=Arbitrary discrete  minUnid=1  maxUnid=16  numValueUnid=5  valueVecDisc=[1 2 3 4]  probVecDisc=[.25 .25 .25 .25]  Seed=SEED+500
  Enabled Gate : EnabledGate
  Entity Departure Event to Function-Call Event : EntityDepartureFunctionCallGenerator
  Entity Sink : EntitySink
  Entity Sink1 : EntitySink
  Entity Sink2 : EntitySink
  Generator 1 : TimeBasedEntityGenerator  Distribution=Exponential  Period=.1  InitialSeed=SEED+10  Maximum=.2  Mean=B  ResponseWhenUnblocked=Delayed restart  EntityType=Standard
  Infinite Server : InfiniteServer  ServiceTime=D  EnableTOPort=on
  Input Switch : InputSwitch  SwitchingCriterion=From signal port p
  Schedule Timeout : ScheduleTimeout  TimeoutInterval=D
  Set Attribute : SetAttribute  AttributeName=DST_X|DST_Y|DST_Z  AttributeFrom=Signal port|Signal port|Signal port  AttributeValue=16|1|1  AttributeTreatAsVector=0|1|1  EvaluatedAttributeValue={ [];[];[]}
      settings: InputPortMap=u0,u1,u2
  Start Timer : StartTimer  TimerTag=Departure
  Time-Based Entity Generator : TimeBasedEntityGenerator  Distribution=Exponential  Period=15  InitialSeed=12731  Maximum=2  Mean=A  PriorityEntityGeneration=350  EntityType=Standard
  Time-Based Entity Generator1 : TimeBasedEntityGenerator  Period=REGULAR
  Time-Based Entity Generator2 : TimeBasedEntityGenerator  Distribution=Uniform  InitialSeed=15948  Minimum=MINU  Maximum=MAXU
  Data_out : PMIOPort  Port=1  Side=Right
  Data_in : PMIOPort  Port=2  Side=Left
  wires:
  Create Generator Selection Variable/1(Out1) -> Enabled Gate/1
  Entity Departure Event to Function-Call Event/1 -> Create Generator Selection Variable/Trigger
  Constant/1 -> Input Switch/1
  DST/1 -> Set Attribute/1
  DST1/1 -> Set Attribute/2
  DST2/1 -> Set Attribute/3
  connections:
  Entity Departure Event to Function-Call Event/RConn1 -- Entity Sink/LConn1
  Time-Based Entity Generator/RConn1 -- Entity Departure Event to Function-Call Event/LConn1
  Generator 1/RConn1 -- Enabled Gate/LConn1
  Time-Based Entity Generator1/RConn1 -- Input Switch/LConn1
  Input Switch/LConn2 -- Time-Based Entity Generator2/RConn1
  Enabled Gate/RConn1 -- Input Switch/LConn3
  Schedule Timeout/LConn1 -- Set Attribute/RConn1
  Cancel Timeout/LConn1 -- Infinite Server/RConn1
  Set Attribute/LConn1 -- Input Switch/RConn1
  Data_out/RConn1 -- Start Timer/RConn1
  Start Timer/LConn1 -- Cancel Timeout/RConn1
  Entity Sink1/LConn1 -- Data_in/RConn1
  Schedule Timeout/RConn1 -- Infinite Server/LConn1
  Infinite Server/RConn2 -- Entity Sink2/LConn1
